simulink model "ADCRawToIab"  (R2020b)
settings: Solver=FixedStepDiscrete  StartTime=0.0  StopTime=100  FixedStep=250*Ts  RelTol=1e-3
values from neighbouring files (symbols this model uses):
  ADC_V_OUT = 0.0 0.00080566640599999992 0.0016113328119999998 0.002416999218 0.0032226656239999997 0.00402833203 0.004833998436 0.0056396648419999992 0.0064453312479999993 0.007250997654 0.00805666406 0.0088623304659999989 0.009667996872 0.010473663278 0.011279329683999998 0.01208499609 0.012890662495999999 0.013696328902 0.014501995308 0.015307661714 0.01611332812 0.016918994525999997 0.017724660931999998 0.0    [ADCRawToIab.sldd]
  DRV_GAIN = 10.0    [ADCRawToIab.sldd]
  DRV_SHUNTR_OHM = 0.007    [ADCRawToIab.sldd]
  DRV_V_REF_Div2 = 1.65    [ADCRawToIab.sldd]
settings Model: DataDictionary=ADCRawToIab.sldd  Creator=unix  LastModifiedBy=unix
settings SolverCC: AutoInsertRateTranBlk=on
settings DataIOCC: SaveOutput=off  SaveTime=off
settings OptimizationCC: DefaultParameterBehavior=Inlined  EnhancedBackFolding=on  PassReuseOutputArgsAs=Individual arguments  ZeroExternalMemoryAtStartup=off  ZeroInternalMemoryAtStartup=off  OptimizeBlockOrder=speed  DifferentSizesBufferReuse=on  OptimizationCustomize=off  EfficientTunableParamExpr=on
settings DebuggingCC: SignalInfNanChecking=warning  SignalRangeChecking=warning  CheckMatrixSingularityMsg=warning  ParameterOverflowMsg=warning  ParameterUnderflowMsg=warning  ParameterPrecisionLossMsg=none  ParameterTunabilityLossMsg=error  UnderSpecifiedDataTypeMsg=warning
settings SFSimCC: MATLABDynamicMemAlloc=off
settings RTWCC: Description=Embedded Coder  SystemTargetFile=ert.tlc  GenCodeOnly=on  TemplateMakefile=ert_default_tmf  GenerateReport=on  IncludeHyperlinkInReport=on  LaunchReport=on  GenerateTraceInfo=on  GenerateTraceReport=on  GenerateTraceReportSl=on  GenerateTraceReportSf=on  GenerateTraceReportEml=on
settings CodeAppCC: ForceParamTrailComments=on  IgnoreCustomStorageClasses=off  OperatorAnnotations=on  SimulinkDataObjDesc=on  SFDataObjDesc=on  InsertBlockDesc=on
settings ERTTargetCC: TargetLangStandard=C99 (ISO)  GenerateSampleERTMain=on  InlinedParameterPlacement=NonHierarchical  ERTCustomFileTemplate=example_file_process.tlc

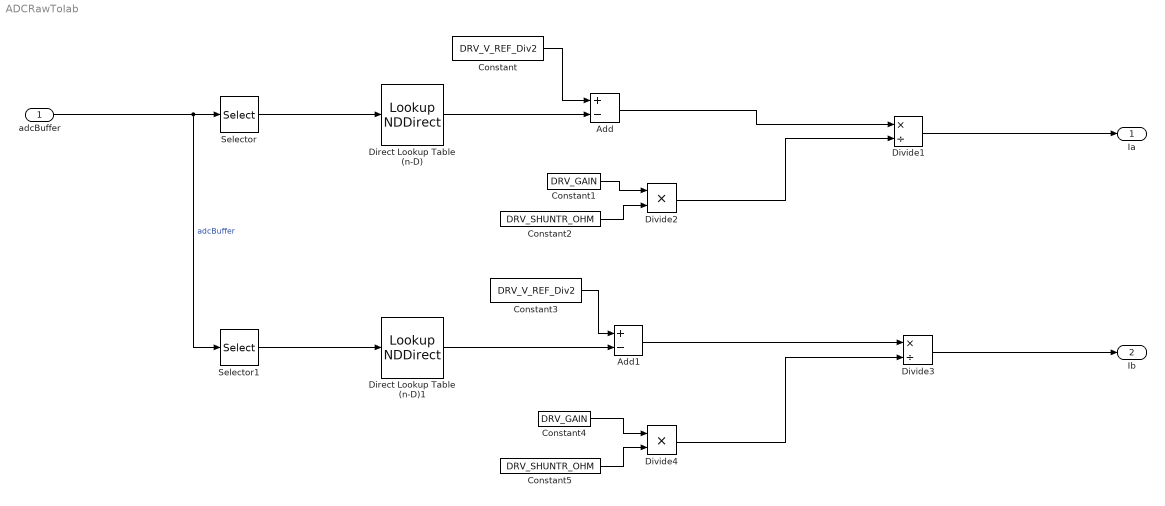
== system ADCRawToIab ==
  adcBuffer : Inport
  Add : Sum  Inputs=+-
  Add1 : Sum  Inputs=+-
  Constant : Constant  Value=DRV_V_REF_Div2
  Constant1 : Constant  Value=DRV_GAIN
  Constant2 : Constant  Value=DRV_SHUNTR_OHM
  Constant3 : Constant  Value=DRV_V_REF_Div2
  Constant4 : Constant  Value=DRV_GAIN
  Constant5 : Constant  Value=DRV_SHUNTR_OHM
  Direct Lookup Table (n-D) : LookupNDDirect  NumberOfTableDimensions=1  Table=ADC_V_OUT
  Direct Lookup Table (n-D)1 : LookupNDDirect  NumberOfTableDimensions=1  Table=ADC_V_OUT
  Divide1 : Product  Inputs=*/  OutMin=0  OutMax=3.3  OutDataTypeStr=fixdt(1,16,2^-8,0)  SaturateOnIntegerOverflow=on
  Divide2 : Product  Inputs=**  OutMin=0  OutMax=3.3  OutDataTypeStr=fixdt(1,16,2^-10,0)  SaturateOnIntegerOverflow=on
  Divide3 : Product  Inputs=*/  OutMin=0  OutMax=3.3  OutDataTypeStr=fixdt(1,16,2^-8,0)  SaturateOnIntegerOverflow=on
  Divide4 : Product  Inputs=**  OutMin=0  OutMax=3.3  OutDataTypeStr=fixdt(1,16,2^-10,0)  SaturateOnIntegerOverflow=on
  Selector : Selector  InputPortWidth=2  IndexOptions=Index vector (dialog)  Indices=1  OutputSizes=1
  Selector1 : Selector  InputPortWidth=2  IndexOptions=Index vector (dialog)  Indices=2  OutputSizes=1
  Ia : Outport  OutDataTypeStr=fixdt(1,16,8)  PortDimensions=1
  Ib : Outport  Port=2  OutDataTypeStr=fixdt(1,16,8)  PortDimensions=1
  wires:
  adcBuffer/1 -> Selector/1, Selector1/1  "adcBuffer"
  Constant2/1 -> Divide2/2
  Selector/1 -> Direct Lookup Table (n-D)/1
  Divide1/1 -> Ia/1
  Constant1/1 -> Divide2/1
  Divide2/1 -> Divide1/2
  Constant/1 -> Add/1
  Direct Lookup Table (n-D)/1 -> Add/2
  Add/1 -> Divide1/1
  Add1/1 -> Divide3/1
  Direct Lookup Table (n-D)1/1 -> Add1/2
  Constant3/1 -> Add1/1
  Divide4/1 -> Divide3/2
  Constant4/1 -> Divide4/1
  Divide3/1 -> Ib/1
  Selector1/1 -> Direct Lookup Table (n-D)1/1
  Constant5/1 -> Divide4/2
